simulink model "knock0"  (Simulink 8.2)
settings: Solver=FixedStepDiscrete  StartTime=0.0  StopTime=10000  FixedStep=1  RelTol=1e-3
values from neighbouring files (symbols this model uses):
  advanceGain = m1*Delta    (= 0.015)    [plotDriver.m]
  initialSpark = 1.6    [plotDriver.m]
  knockGenP = myPcurve1    [plotDriver.m]
  knockGenTheta = theta    [plotDriver.m]
  retardGain = m2*Delta    (= 1.485)    [plotDriver.m]
settings Model: Creator=jpeytonj  LastModifiedBy=jpeytonj
settings DataIOCC: LimitDataPoints=off  SaveFormat=Structure
settings OptimizationCC: ExpressionDepthLimit=128  InitFltsAndDblsToZero=on
settings DebuggingCC: SaveWithParameterizedLinksMsg=none  SignalResolutionControl=TryResolveAllWithWarning  MultiTaskDSMMsg=warning  MultiTaskCondExecSysMsg=none  StateNameClashWarn=none
settings SFSimCC: SimParseCustomCode=off
settings RTWCC: IncludeERTFirstTime=on
settings GRTTargetCC: TargetFcnLib=ansi_tfl_tmw.mat

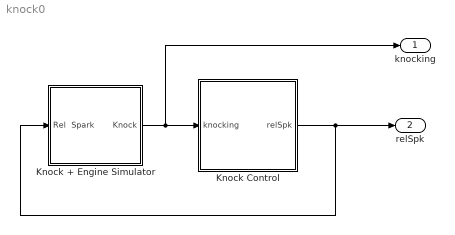
== system knock0 ==
  Knock + Engine Simulator : Subsystem
  Knock Control : Subsystem  TreatAsAtomicUnit=on  mask{initialSpark=initialSpark, retardGain=retardGain, advanceGain=advanceGain, p=0, spkMin=-3, spkMax=2, hiThreshold=2, loThreshold=-2}
      mask prompts: retardGain "Retard Gain:"; advanceGain "Advance Gain:"; p "Desired Knock Probability:"; spkMin "Lower Saturation Limit:"; spkMax "Upper Saturation Limit"; hiThreshold "CumSum Hi Threshold:"; loThreshold "CumSum Lo Threshold:"
  knocking : Outport
  relSpk : Outport  Port=2
  wires:
  Knock + Engine Simulator/1(Knock) -> Knock Control/1(knocking), knocking/1
  Knock Control/1(relSpk) -> Knock + Engine Simulator/1(Rel  Spark), relSpk/1

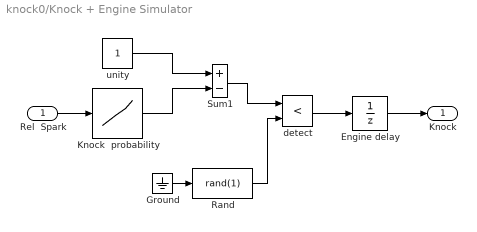
== system knock0/Knock + Engine Simulator ==
  Rel  Spark : Inport
  Engine delay : UnitDelay
  Ground : Ground
  Knock  probability : Lookup  InputValues=knockGenTheta  Table=knockGenP
  Rand : MATLABFcn  MATLABFcn=rand(1)  OutputDimensions=1  SampleTime=[1 0]
  Sum1 : Sum  Inputs=+-
  detect : RelationalOperator  Operator=<  OutDataTypeStr=boolean
  unity : Constant
  Knock : Outport
  wires:
  unity/1 -> Sum1/1
  Knock  probability/1 -> Sum1/2
  Sum1/1 -> detect/1
  Rel  Spark/1 -> Knock  probability/1
  detect/1 -> Engine delay/1
  Engine delay/1 -> Knock/1
  Rand/1 -> detect/2
  Ground/1 -> Rand/1

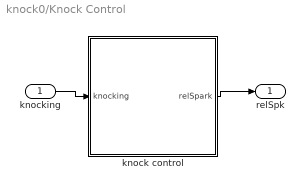
== system knock0/Knock Control ==
  knocking : Inport
  knock control : MATLAB Function  TreatAsAtomicUnit=on
  relSpk : Outport
  wires:
  knock control/1(relSpark) -> relSpk/1
  knocking/1 -> knock control/1(knocking)

== matlab function Knock Control/knock control ==
  data: knocking input double; initialSpark parameter double; relSpark output double; retardGain parameter double; advanceGain parameter double; spkMin parameter double; spkMax parameter double
function relSpark = knCtrl(knocking,initialSpark,retardGain,advanceGain,spkMin,spkMax)

%Computes the new relative spark angle (deg) based on:
%   knocking:       a boolean knock signal
%   initialSpark:   the initial spark relative to borderline
%   retardGain:     the retard amount (deg)
%   advanceGain     the advance amount (deg)

%   Copyright 2009 Villanova University
%   Author: James C. Peyton Jones  (5/1/2009)
%   Version knock0:  Traditional Knock Control
%   Revision:        Date:
%
%

%Declare persistent variables
persistent relSpk

%Initialization
if isempty(relSpk),
    relSpk= double(initialSpark);
end;

%Traditional knock control
if knocking,
	relSpk= relSpk - retardGain;
else
	relSpk= relSpk + advanceGain;
end;

%Apply saturation limits
if relSpk>spkMax, relSpk=spkMax; end;
if relSpk<spkMin, relSpk=spkMin; end;

%Output value
relSpark= double(relSpk);
